simulink model "Q9"  (R2020b)
settings: Solver=FixedStepAuto  StartTime=0.0  StopTime=10  FixedStep=0.01  RelTol=1e-3
settings Model: Creator=AKSHAY JP PAWAR  LastModifiedBy=AKSHAY JP PAWAR
settings DebuggingCC: ArithmeticOperatorsInVariantConditions=warning
settings SFSimCC: CustomCodeUndefinedFunction=UseInterfaceOnly
settings CodeAppCC: StateflowObjectComments=on

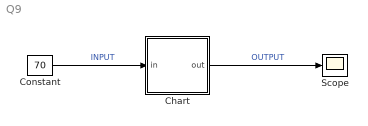
== system Q9 ==
  Chart : Stateflow chart  TreatAsAtomicUnit=on
  Constant : Constant  Value=70
  Scope : Scope
  wires:
  Chart/1(out) -> Scope/1  "OUTPUT"
  Constant/1 -> Chart/1(in)  "INPUT"

== stateflow chart Q9/Chart ==
  state N1
    entry:
    out=1;
    i=1;
    during:
    i=i+1;
  state N2
    entry:
    out=0;
    during:
    i=i+1;
  (default) -> N1
  N1 -> N2 : [i>=in]
  N2 -> N1 : [i>=100]
  data: out output double; i local double; in input double
